simulink model "TestQ"  (R2018b)
settings: Solver=VariableStepAuto  StartTime=0.0  StopTime=tSimEnd  MaxStep=0.001  RelTol=1e-3  EnableMultiTasking=on
InitFcn:
  | clear
  | load 2017-07-18-13-36-00_fullrate_back_forth.mat
  | if ~exist( 'logOriginal' )
  |     logOriginal = dataInOriginal
  | end
  | flog = logOriginal;
  | tSart = flog.vehicle_attitude.time(1);
  | timeStep = 0; % flog.vehicle_attitude.time(2) - flog.vehicle_attitude.time(1);
  | flog.sensor_combined.time = flog.sensor_combined.time - flog.vehicle_attitude.time(1) - timeStep;
  | flog.att_pos_mocap.time = flog.att_pos_mocap.time - flog.vehicle_attitude.time(1) - timeStep;
  | flog.control_state.time = flog.control_state.time - flog.vehicle_attitude.time(1) - timeStep;
  | flog.vehicle_global_position.time = flog.vehicle_global_position.time - flog.vehicle_attitude.time(1) - timeStep;
  | flog.vehicle_attitude.time = flog.vehicle_attitude.time - flog.vehicle_attitude.time(1);
  | 
  | tSimEnd = flog.vehicle_attitude.time(end);
libraries: simulink_extras x3
(part 1 of 2)
settings Model: Creator=jban039  LastModifiedBy=jban039
settings DataIOCC: LimitDataPoints=on
settings OptimizationCC: LifeSpan=inf
settings DebuggingCC: AllowSymbolicDim=off  SFUnexpectedBacktrackingDiag=warning  SFNoUnconditionalDefaultTransitionDiag=warning  SFExecutionAtInitializationDiag=none
settings ModelReferenceCC: PropagateSignalLabelsOutOfModel=off
settings SFSimCC: SimUseLocalCustomCode=off
settings RTWCC: RTWUseLocalCustomCode=off
settings CodeAppCC: StateflowObjectComments=on
settings GRTTargetCC: TargetLangStandard=C89/C90 (ANSI)
settings ConfigComp: CovMetricSettings=dw  CovHtmlReporting=on  CovSaveCumulativeToWorkspaceVar=on  CovSaveSingleToWorkspaceVar=on  CovExternalEMLEnable=off

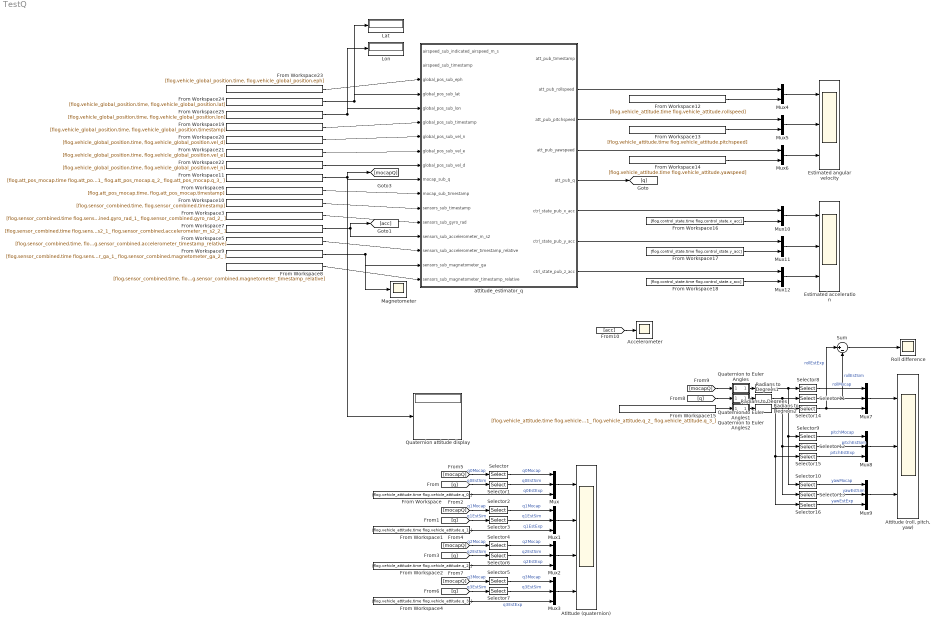
== system TestQ ==
  Accelerometer : Scope
  Atittude (quaternion) : Scope  NumInputPorts=4
  "Attitude (roll, pitch, yaw)" : Scope  NumInputPorts=3
  Estimated acceleration : Scope  NumInputPorts=3
  Estimated angular velocity : Scope  NumInputPorts=3
  From Workspace : FromWorkspace  VariableName=[flog.vehicle_attitude.time flog.vehicle_attitude.q_0_]  SampleTime=0  Interpolate=off  OutputAfterFinalValue=Holding final value
  From Workspace1 : FromWorkspace  VariableName=[flog.vehicle_attitude.time flog.vehicle_attitude.q_1_]  SampleTime=0  Interpolate=off  OutputAfterFinalValue=Holding final value
  From Workspace10 : FromWorkspace  VariableName=[flog.sensor_combined.time, flog.sensor_combined.timestamp]  SampleTime=0  Interpolate=off  OutputAfterFinalValue=Holding final value
  From Workspace11 : FromWorkspace  VariableName=[flog.att_pos_mocap.time flog.att_pos_mocap.q_0_ flog.att_pos_mocap.q_1_ flog.att_pos_mocap.q_2_ flog.att_pos_mocap.q_3_ ]  SampleTime=0  Interpolate=off  OutputAfterFinalValue=Holding final value
  From Workspace12 : FromWorkspace  VariableName=[flog.vehicle_attitude.time flog.vehicle_attitude.rollspeed]  SampleTime=0  Interpolate=off  OutputAfterFinalValue=Holding final value
  From Workspace13 : FromWorkspace  VariableName=[flog.vehicle_attitude.time flog.vehicle_attitude.pitchspeed]  SampleTime=0  Interpolate=off  OutputAfterFinalValue=Holding final value
  From Workspace14 : FromWorkspace  VariableName=[flog.vehicle_attitude.time flog.vehicle_attitude.yawspeed]  SampleTime=0  Interpolate=off  OutputAfterFinalValue=Holding final value
  From Workspace15 : FromWorkspace  VariableName=[flog.vehicle_attitude.time flog.vehicle_attitude.q_0_ flog.vehicle_attitude.q_1_ flog.vehicle_attitude.q_2_ flog.vehicle_attitude.q_3_]  SampleTime=0  Interpolate=off  OutputAfterFinalValue=Holding final value
  From Workspace16 : FromWorkspace  VariableName=[flog.control_state.time flog.control_state.x_acc]  SampleTime=0  Interpolate=off  OutputAfterFinalValue=Holding final value
  From Workspace17 : FromWorkspace  VariableName=[flog.control_state.time flog.control_state.y_acc]  SampleTime=0  Interpolate=off  OutputAfterFinalValue=Holding final value
  From Workspace18 : FromWorkspace  VariableName=[flog.control_state.time flog.control_state.z_acc]  SampleTime=0  Interpolate=off  OutputAfterFinalValue=Holding final value
  From Workspace19 : FromWorkspace  VariableName=[flog.vehicle_global_position.time, flog.vehicle_global_position.timestamp]  SampleTime=0  Interpolate=off  OutputAfterFinalValue=Holding final value
  From Workspace2 : FromWorkspace  VariableName=[flog.vehicle_attitude.time flog.vehicle_attitude.q_2_]  SampleTime=0  Interpolate=off  OutputAfterFinalValue=Holding final value
  From Workspace20 : FromWorkspace  VariableName=[flog.vehicle_global_position.time, flog.vehicle_global_position.vel_d]  SampleTime=0  Interpolate=off  OutputAfterFinalValue=Holding final value
  From Workspace21 : FromWorkspace  VariableName=[flog.vehicle_global_position.time, flog.vehicle_global_position.vel_e]  SampleTime=0  Interpolate=off  OutputAfterFinalValue=Holding final value
  From Workspace22 : FromWorkspace  VariableName=[flog.vehicle_global_position.time, flog.vehicle_global_position.vel_n]  SampleTime=0  Interpolate=off  OutputAfterFinalValue=Holding final value
  From Workspace23 : FromWorkspace  VariableName=[flog.vehicle_global_position.time, flog.vehicle_global_position.eph]  SampleTime=0  Interpolate=off  OutputAfterFinalValue=Holding final value
  From Workspace24 : FromWorkspace  VariableName=[flog.vehicle_global_position.time, flog.vehicle_global_position.lat]  SampleTime=0  Interpolate=off  OutputAfterFinalValue=Holding final value
  From Workspace25 : FromWorkspace  VariableName=[flog.vehicle_global_position.time, flog.vehicle_global_position.lon]  SampleTime=0  Interpolate=off  OutputAfterFinalValue=Holding final value
  From Workspace3 : FromWorkspace  VariableName=[flog.sensor_combined.time flog.sensor_combined.gyro_rad_0_ flog.sensor_combined.gyro_rad_1_ flog.sensor_combined.gyro_rad_2_ ]  SampleTime=0  Interpolate=off  OutputAfterFinalValue=Holding final value
  From Workspace4 : FromWorkspace  VariableName=[flog.vehicle_attitude.time flog.vehicle_attitude.q_3_]  SampleTime=0  Interpolate=off  OutputAfterFinalValue=Holding final value
  From Workspace5 : FromWorkspace  VariableName=[flog.sensor_combined.time, flog.sensor_combined.accelerometer_timestamp_relative]  SampleTime=0  Interpolate=off  OutputAfterFinalValue=Holding final value
  From Workspace6 : FromWorkspace  VariableName=[flog.att_pos_mocap.time, flog.att_pos_mocap.timestamp]  SampleTime=0  Interpolate=off  OutputAfterFinalValue=Holding final value
  From Workspace7 : FromWorkspace  VariableName=[flog.sensor_combined.time flog.sensor_combined.accelerometer_m_s2_0_ flog.sensor_combined.accelerometer_m_s2_1_ flog.sensor_combined.accelerometer_m_s2_2_ ]  SampleTime=0  Interpolate=off  OutputAfterFinalValue=Holding final value
  From Workspace8 : FromWorkspace  VariableName=[flog.sensor_combined.time, flog.sensor_combined.magnetometer_timestamp_relative]  SampleTime=0  Interpolate=off  OutputAfterFinalValue=Holding final value
  From Workspace9 : FromWorkspace  VariableName=[flog.sensor_combined.time flog.sensor_combined.magnetometer_ga_0_ flog.sensor_combined.magnetometer_ga_1_ flog.sensor_combined.magnetometer_ga_2_ ]  SampleTime=0  Interpolate=off  OutputAfterFinalValue=Holding final value
  Lat : Display
  Lon : Display
  Magnetometer : Scope
  Mux{,1..3,7..9} (7 alike) : Mux  Inputs=3
  Mux{4..6,10..12} (6 alike) : Mux  Inputs=2
  Quaternion to Euler Angles : Subsystem  AncestorBlock=QuaternionLibrary/Quaternion to Euler Angles
      mask help: Convert an orientation quaternion to a vector of Euler angles
      mask Help:
      | Convert an orientation quaternion
      | [q1 q2 q3 q4]
      | where:
      | - q1 is the rotation in radians
      | - [q2 q3 q4] is the vector around which the rotation is performed)
      | to a vector of Euler angles
      | [roll, pitch, yaw]
      | Based on code from the PX4 firmware: https://github.com/PX4/Firmware
      mask Display: disp('Q2E')
  Quaternion to Euler Angles1 : Subsystem  AncestorBlock=QuaternionLibrary/Quaternion to Euler Angles
      mask help: Convert an orientation quaternion to a vector of Euler angles
      mask Help:
      | Convert an orientation quaternion
      | [q1 q2 q3 q4]
      | where:
      | - q1 is the rotation in radians
      | - [q2 q3 q4] is the vector around which the rotation is performed)
      | to a vector of Euler angles
      | [roll, pitch, yaw]
      | Based on code from the PX4 firmware: https://github.com/PX4/Firmware
      mask Display: disp('Q2E')
  Quaternion to Euler Angles2 : Subsystem  AncestorBlock=QuaternionLibrary/Quaternion to Euler Angles
      mask help: Convert an orientation quaternion to a vector of Euler angles
      mask Help:
      | Convert an orientation quaternion
      | [q1 q2 q3 q4]
      | where:
      | - q1 is the rotation in radians
      | - [q2 q3 q4] is the vector around which the rotation is performed)
      | to a vector of Euler angles
      | [roll, pitch, yaw]
      | Based on code from the PX4 firmware: https://github.com/PX4/Firmware
      mask Display: disp('Q2E')
  Quaternion attitude display : Display
  Radians to Degrees : simulink_extras/Transformations/Radians to Degrees
  Radians to Degrees1 : simulink_extras/Transformations/Radians to Degrees
  Radians to Degrees2 : simulink_extras/Transformations/Radians to Degrees
  Roll difference : Scope
  Selector : Selector  InputPortWidth=4  IndexOptions=Index vector (dialog)  Indices=[1]  OutputSizes=1
  Selector1 : Selector  InputPortWidth=4  IndexOptions=Index vector (dialog)  Indices=[1]  OutputSizes=1
  Selector10 : Selector  InputPortWidth=3  IndexOptions=Index vector (dialog)  Indices=3  OutputSizes=1
  Selector{8..9,11..12,14..15} (6 alike) : Selector  InputPortWidth=3  IndexOptions=Index vector (dialog)  Indices=[1]  OutputSizes=1
  Selector13 : Selector  InputPortWidth=3  IndexOptions=Index vector (dialog)  Indices=3  OutputSizes=1
  Selector16 : Selector  InputPortWidth=3  IndexOptions=Index vector (dialog)  Indices=3  OutputSizes=1
  Selector2 : Selector  InputPortWidth=4  IndexOptions=Index vector (dialog)  Indices=2  OutputSizes=1
  Selector3 : Selector  InputPortWidth=4  IndexOptions=Index vector (dialog)  Indices=2  OutputSizes=1
  Selector4 : Selector  InputPortWidth=4  IndexOptions=Index vector (dialog)  Indices=3  OutputSizes=1
  Selector5 : Selector  InputPortWidth=4  IndexOptions=Index vector (dialog)  Indices=4  OutputSizes=1
  Selector6 : Selector  InputPortWidth=4  IndexOptions=Index vector (dialog)  Indices=3  OutputSizes=1
  Selector7 : Selector  InputPortWidth=4  IndexOptions=Index vector (dialog)  Indices=4  OutputSizes=1
  Sum : Sum  Inputs=|+-
  attitude_estimator_q : Subsystem  AncestorBlock=Px4Library/attitude_estimator_q  mask(PX4 LPE (local position estimator): local_position_estimator){Q_SAMPLING_PERIOD=1/250, INIT_Q=[-0.726717000000000,-0.00744072000000000,-0.00534285000000000,-0.686876000000000]', ATT_W_ACC=0.2, ATT_W_MAG=0.1, ATT_W_EXT_HDG=0.1, ATT_W_GYRO_BIAS=0.1, ATT_MAG_DECL=0.0, ATT_MAG_DECL_A=1, ATT_EXT_HDG_M=2, ATT_ACC_COMP=1, ATT_BIAS_MAX=0.05, FW_ARSP_MODE=0}
      mask prompts: Q_SAMPLING_PERIOD "Sampling period (s)"; INIT_Q "INIT_Q - Initial UAV orientation - set to 0 to let controller decide (bugged) (-)"; ATT_W_ACC "ATT_W_ACC - Complimentary filter accelerometer weight (-)"; ATT_W_MAG "ATT_W_MAG - Complimentary filter magnetometer weight (-)"; ATT_W_EXT_HDG "ATT_W_EXT_HDG - Complimentary filter external heading weight (-)"; ATT_W_GYRO_BIAS "ATT_W_GYRO_BIAS - Complimentary filter gyroscope bias weight (-)"; ATT_MAG_DECL "ATT_MAG_DECL - Magnetic declination. Not used when GPS available (deg)"; ATT_MAG_DECL_A "ATT_MAG_DECL_A - Automatic GPS based declination compensation (-)"; ATT_EXT_HDG_M "ATT_EXT_HDG_M - External heading usage mode (from Motion capture/Vision) (-), 0 None 1 Vision 2 Motion Capture"; ATT_ACC_COMP "ATT_ACC_COMP - Acceleration compensation based on GPS velocity. (-)"; ATT_BIAS_MAX "ATT_BIAS_MAX - Gyro bias limit (rad/s)"; FW_ARSP_MODE "FW_ARSP_MODE - Method used to publish the airspeed (-), 0 Measured airspeed 1 Vehicle ground speed 2 Airspeed invalid"
      mask TypeOptions ATT_EXT_HDG_M: 0 | 1 | 2
      mask TypeOptions FW_ARSP_MODE: 0 | 1 | 2
  wires:
  Mux1/1 -> Atittude (quaternion)/2
  Mux/1 -> Atittude (quaternion)/1
  Mux2/1 -> Atittude (quaternion)/3
  attitude_estimator_q/5(att_pub_q) -> [q]
  From Workspace/1 -> Mux/3  "q0EstExp"
  Selector1/1 -> Mux/2  "q0EstSim"
  From Workspace11/1 -> Quaternion attitude display/1, [mocapQ], attitude_estimator_q/10(mocap_sub_q)
  From Workspace6/1 -> attitude_estimator_q/11(mocap_sub_timestamp)
  Selector/1 -> Mux/1  "q0Mocap"
  From Workspace7/1 -> attitude_estimator_q/14(sensors_sub_accelerometer_m_s2), [acc]
  From Workspace9/1 -> attitude_estimator_q/16(sensors_sub_magnetometer_ga), Magnetometer/1
  From Workspace3/1 -> attitude_estimator_q/13(sensors_sub_gyro_rad)
  From Workspace1/1 -> Mux1/3  "q1EstExp"
  Selector3/1 -> Mux1/2  "q1EstSim"
  Selector2/1 -> Mux1/1  "q1Mocap"
  From Workspace2/1 -> Mux2/3  "q2EstExp"
  Selector6/1 -> Mux2/2  "q2EstSim"
  Selector4/1 -> Mux2/1  "q2Mocap"
  Mux3/1 -> Atittude (quaternion)/4
  From Workspace4/1 -> Mux3/3  "q3EstExp"
  Selector7/1 -> Mux3/2  "q3EstSim"
  Selector5/1 -> Mux3/1  "q3Mocap"
  [mocapQ] -> Selector/1  "q0Mocap"
  [q] -> Selector1/1  "q0EstSim"
  [mocapQ] -> Selector2/1  "q1Mocap"
  [q] -> Selector3/1  "q1EstSim"
  [mocapQ] -> Selector4/1  "q2Mocap"
  [q] -> Selector6/1  "q2EstSim"
  [mocapQ] -> Selector5/1  "q3Mocap"
  [q] -> Selector7/1  "q3EstSim"
  From Workspace8/1 -> attitude_estimator_q/17(sensors_sub_magnetometer_timestamp_relative)
  From Workspace5/1 -> attitude_estimator_q/15(sensors_sub_accelerometer_timestamp_relative)
  Mux4/1 -> Estimated angular velocity/1
  Mux5/1 -> Estimated angular velocity/2
  Mux6/1 -> Estimated angular velocity/3
  attitude_estimator_q/2(att_pub_rollspeed) -> Mux4/1
  attitude_estimator_q/3(att_pub_pitchspeed) -> Mux5/1
  attitude_estimator_q/4(att_pub_yawspeed) -> Mux6/1
  From Workspace12/1 -> Mux4/2
  From Workspace13/1 -> Mux5/2
  From Workspace14/1 -> Mux6/2
  Quaternion to Euler Angles/1(euler) -> Radians to Degrees/1
  Quaternion to Euler Angles1/1(euler) -> Radians to Degrees1/1
  Mux7/1 -> "Attitude (roll, pitch, yaw)"/1
  Mux8/1 -> "Attitude (roll, pitch, yaw)"/2
  Mux9/1 -> "Attitude (roll, pitch, yaw)"/3
  Selector8/1 -> Mux7/1  "rollMocap"
  Selector11/1 -> Sum/2, Mux7/2  "rollEstSim"
  Selector9/1 -> Mux8/1  "pitchMocap"
  Selector12/1 -> Mux8/2  "pitchEstSim"
  Selector13/1 -> Mux9/2  "yawEstSim"
  Selector10/1 -> Mux9/1  "yawMocap"
  [mocapQ] -> Quaternion to Euler Angles/1(quaternion)
  [q] -> Quaternion to Euler Angles1/1(quaternion)
  From Workspace15/1 -> Quaternion to Euler Angles2/1(quaternion)
  Selector16/1 -> Mux9/3  "yawEstExp"
  Selector15/1 -> Mux8/3  "pitchEstExp"
  Selector14/1 -> Sum/1, Mux7/3  "rollEstExp"
  Radians to Degrees2/1 -> Selector16/1, Selector15/1, Selector14/1
  Radians to Degrees/1 -> Selector10/1, Selector9/1, Selector8/1
  Radians to Degrees1/1 -> Selector13/1, Selector12/1, Selector11/1
  Quaternion to Euler Angles2/1(euler) -> Radians to Degrees2/1
  Sum/1 -> Roll difference/1
  Mux10/1 -> Estimated acceleration/1
  Mux11/1 -> Estimated acceleration/2
  Mux12/1 -> Estimated acceleration/3
  attitude_estimator_q/6(ctrl_state_pub_x_acc) -> Mux10/1
  attitude_estimator_q/7(ctrl_state_pub_y_acc) -> Mux11/1
  attitude_estimator_q/8(ctrl_state_pub_z_acc) -> Mux12/1
  From Workspace16/1 -> Mux10/2
  From Workspace17/1 -> Mux11/2
  From Workspace18/1 -> Mux12/2
  From Workspace10/1 -> attitude_estimator_q/12(sensors_sub_timestamp)
  From Workspace20/1 -> attitude_estimator_q/7(global_pos_sub_vel_n)
  From Workspace19/1 -> attitude_estimator_q/6(global_pos_sub_timestamp)
  From Workspace21/1 -> attitude_estimator_q/8(global_pos_sub_vel_e)
  From Workspace22/1 -> attitude_estimator_q/9(global_pos_sub_vel_d)
  From Workspace25/1 -> attitude_estimator_q/5(global_pos_sub_lon), Lon/1
  From Workspace24/1 -> attitude_estimator_q/4(global_pos_sub_lat), Lat/1
  From Workspace23/1 -> attitude_estimator_q/3(global_pos_sub_eph)
  [acc] -> Accelerometer/1

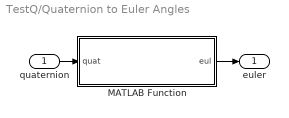
== system TestQ/Quaternion to Euler Angles ==
  quaternion : Inport
  MATLAB Function : MATLAB Function  TreatAsAtomicUnit=on
  euler : Outport
  wires:
  quaternion/1 -> MATLAB Function/1(quat)
  MATLAB Function/1(eul) -> euler/1

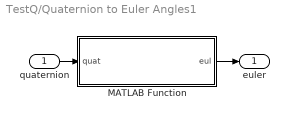
== system TestQ/Quaternion to Euler Angles1 ==
  quaternion : Inport
  MATLAB Function : MATLAB Function  TreatAsAtomicUnit=on
  euler : Outport
  wires:
  quaternion/1 -> MATLAB Function/1(quat)
  MATLAB Function/1(eul) -> euler/1

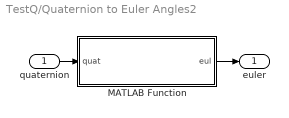
== system TestQ/Quaternion to Euler Angles2 ==
  quaternion : Inport
  MATLAB Function : MATLAB Function  TreatAsAtomicUnit=on
  euler : Outport
  wires:
  quaternion/1 -> MATLAB Function/1(quat)
  MATLAB Function/1(eul) -> euler/1

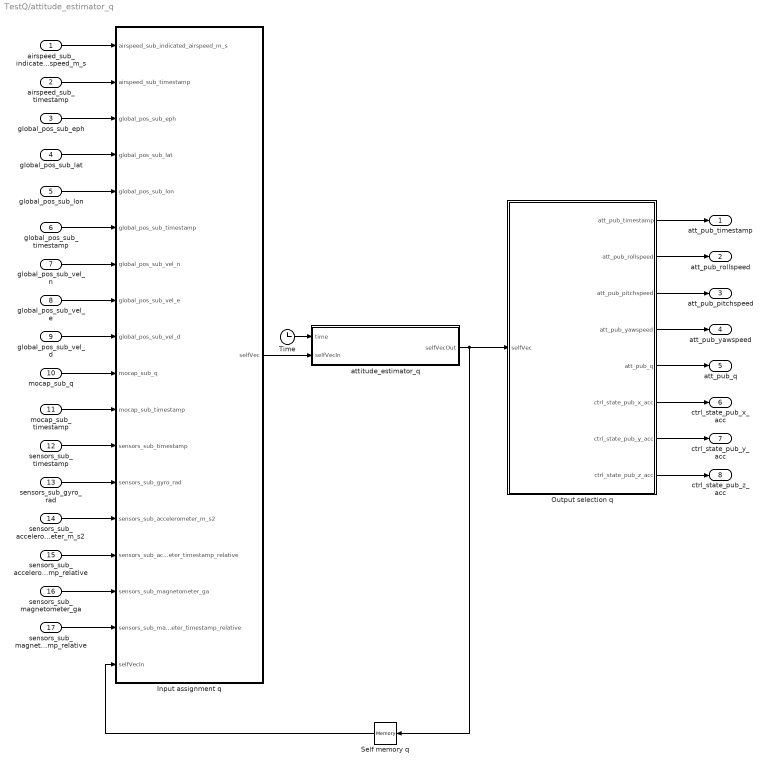
== system TestQ/attitude_estimator_q ==
  airspeed_sub_indicated_airspeed_m_s : Inport
  airspeed_sub_timestamp : Inport  Port=2
  global_pos_sub_eph : Inport  Port=3
  global_pos_sub_lat : Inport  Port=4
  global_pos_sub_lon : Inport  Port=5
  global_pos_sub_timestamp : Inport  Port=6
  global_pos_sub_vel_n : Inport  Port=7
  global_pos_sub_vel_e : Inport  Port=8
  global_pos_sub_vel_d : Inport  Port=9
  mocap_sub_q : Inport  Port=10
  mocap_sub_timestamp : Inport  Port=11
  sensors_sub_timestamp : Inport  Port=12
  sensors_sub_gyro_rad : Inport  Port=13
  sensors_sub_accelerometer_m_s2 : Inport  Port=14
  sensors_sub_accelerometer_timestamp_relative : Inport  Port=15
  sensors_sub_magnetometer_ga : Inport  Port=16
  sensors_sub_magnetometer_timestamp_relative : Inport  Port=17
  Input assignment q : MATLAB Function  TreatAsAtomicUnit=on
  Output selection q : MATLAB Function  TreatAsAtomicUnit=on
  Self memory q : Memory  InitialCondition=[ATT_ACC_COMP, 0, 0, 0, 0, 0, 0, 0, FW_ARSP_MODE, 0, 0, 0, 0, 0, 0, 0, 0, INIT_Q(1), INIT_Q(2), INIT_Q(3), INIT_Q(4), ATT_BIAS_MAX, 0, 0, INIT_Q(1), INIT_Q(2), INIT_Q(3), INIT_Q(4), 0, 0, 0, 0, 0, 0, 0, 0, 0, 0, 0, 0, 0.02, 0, ATT_EXT_HDG_M, 0, 0, 0, 0, 0, 0, 0, 0, 0, 0, 0, 0, 0, 0, 0, 0, 0, 0, 0, 0, 0, 0, 0, 0, 0, 0, 0, 0, 0, 0, 0, 0, 0, 0, 0, 0, 0, 0, 0, 0, 0, 0, 0, 0, 0, 0, 0, 0, 0, 0, 0, 0, 0, 0, 0, 0, 0, 0, 0, 0, 0, 0, 0, 0, 0, 0, 0, 0, 0, 0, 0, 0, 0, 0, 0, 0, 0, 0, 0, 0, 0, 0, 0, 0, 0, 0, 0, 0, 0, ATT_MAG_DECL, ATT_MAG_DECL_A, 0, 0, 0, 0, 0, 0, 0, 0, 0, 0, 0, 0, 0, 0, 0, 0, 0, 0, 0, 0, 0, 0, INIT_Q(1), INIT_Q(2), INIT_Q(3), INIT_Q(4), 0, 0, 0, 0, 0, 0, 0, 0, 0, 0, 0, 0, 0, 0, 0, 0, 0, 0, 0, 0, 0, 0, 0, 0, 0, 0, 0, 0, 0, 0, 0, 0, 0, 0, 0, 0, 0, 0, 0, ATT_W_ACC, ATT_W_EXT_HDG, ATT_W_GYRO_BIAS, ATT_W_MAG, 0, 0]
  Time : Clock
  attitude_estimator_q : MATLAB Function  TreatAsAtomicUnit=on  SystemSampleTime=Q_SAMPLING_PERIOD
  att_pub_timestamp : Outport
  att_pub_rollspeed : Outport  Port=2
  att_pub_pitchspeed : Outport  Port=3
  att_pub_yawspeed : Outport  Port=4
  att_pub_q : Outport  Port=5
  ctrl_state_pub_x_acc : Outport  Port=6
  ctrl_state_pub_y_acc : Outport  Port=7
  ctrl_state_pub_z_acc : Outport  Port=8
  wires:
  Output selection q/8(ctrl_state_pub_z_acc) -> ctrl_state_pub_z_acc/1
  Output selection q/7(ctrl_state_pub_y_acc) -> ctrl_state_pub_y_acc/1
  Output selection q/6(ctrl_state_pub_x_acc) -> ctrl_state_pub_x_acc/1
  Output selection q/5(att_pub_q) -> att_pub_q/1
  Output selection q/4(att_pub_yawspeed) -> att_pub_yawspeed/1
  Output selection q/3(att_pub_pitchspeed) -> att_pub_pitchspeed/1
  Output selection q/2(att_pub_rollspeed) -> att_pub_rollspeed/1
  Output selection q/1(att_pub_timestamp) -> att_pub_timestamp/1
  sensors_sub_magnetometer_timestamp_relative/1 -> Input assignment q/17(sensors_sub_magnetometer_timestamp_relative)
  sensors_sub_magnetometer_ga/1 -> Input assignment q/16(sensors_sub_magnetometer_ga)
  sensors_sub_accelerometer_timestamp_relative/1 -> Input assignment q/15(sensors_sub_accelerometer_timestamp_relative)
  sensors_sub_accelerometer_m_s2/1 -> Input assignment q/14(sensors_sub_accelerometer_m_s2)
  sensors_sub_gyro_rad/1 -> Input assignment q/13(sensors_sub_gyro_rad)
  sensors_sub_timestamp/1 -> Input assignment q/12(sensors_sub_timestamp)
  mocap_sub_timestamp/1 -> Input assignment q/11(mocap_sub_timestamp)
  mocap_sub_q/1 -> Input assignment q/10(mocap_sub_q)
  global_pos_sub_vel_d/1 -> Input assignment q/9(global_pos_sub_vel_d)
  global_pos_sub_vel_e/1 -> Input assignment q/8(global_pos_sub_vel_e)
  global_pos_sub_vel_n/1 -> Input assignment q/7(global_pos_sub_vel_n)
  global_pos_sub_timestamp/1 -> Input assignment q/6(global_pos_sub_timestamp)
  global_pos_sub_lon/1 -> Input assignment q/5(global_pos_sub_lon)
  global_pos_sub_lat/1 -> Input assignment q/4(global_pos_sub_lat)
  global_pos_sub_eph/1 -> Input assignment q/3(global_pos_sub_eph)
  airspeed_sub_timestamp/1 -> Input assignment q/2(airspeed_sub_timestamp)
  airspeed_sub_indicated_airspeed_m_s/1 -> Input assignment q/1(airspeed_sub_indicated_airspeed_m_s)
  Time/1 -> attitude_estimator_q/1(time)
  Self memory q/1 -> Input assignment q/18(selfVecIn)
  attitude_estimator_q/1(selfVecOut) -> Self memory q/1, Output selection q/1(selfVec)
  Input assignment q/1(selfVec) -> attitude_estimator_q/2(selfVecIn)

== matlab function TestQ/Quaternion to Euler Angles1/MATLAB Function ==
  data: quat input; eul output
function eul   = QuaternionToEuler( quat )
%QUATERNIONTOEULER Convert quaternion to euler angles
%   Based on PX4 Firmware code: https://github.com/PX4/Firmware
%   Written by:    J.X.J. Bannwarth, 2016/08/29
%   Last modified: J.X.J. Bannwarth, 2018/12/11

    eul = [ atan2(2.0 .* (quat(1) .* quat(2) + quat(3) .* quat(4)), ...
                1.0 - 2.0 .* (quat(2) .* quat(2) + quat(3) .* quat(3)));
	        asin(2.0 .* (quat(1) .* quat(3) - quat(4) .* quat(2)));
            atan2(2.0 .* (quat(1) .* quat(4) + quat(2) .* quat(3)), ...
                1.0 - 2.0 .* (quat(3) .* quat(3) + quat(4) .* quat(4))) ];
end

== matlab function TestQ/Quaternion to Euler Angles/MATLAB Function ==
  data: quat input; eul output
function eul   = QuaternionToEuler( quat )
%QUATERNIONTOEULER Convert quaternion to euler angles
%   Based on PX4 Firmware code: https://github.com/PX4/Firmware
%   Written by:    J.X.J. Bannwarth, 2016/08/29
%   Last modified: J.X.J. Bannwarth, 2018/12/11

    eul = [ atan2(2.0 .* (quat(1) .* quat(2) + quat(3) .* quat(4)), ...
                1.0 - 2.0 .* (quat(2) .* quat(2) + quat(3) .* quat(3)));
	        asin(2.0 .* (quat(1) .* quat(3) - quat(4) .* quat(2)));
            atan2(2.0 .* (quat(1) .* quat(4) + quat(2) .* quat(3)), ...
                1.0 - 2.0 .* (quat(3) .* quat(3) + quat(4) .* quat(4))) ];
end

== matlab function TestQ/Quaternion to Euler Angles2/MATLAB Function ==
  data: quat input; eul output
function eul   = QuaternionToEuler( quat )
%QUATERNIONTOEULER Convert quaternion to euler angles
%   Based on PX4 Firmware code: https://github.com/PX4/Firmware
%   Written by:    J.X.J. Bannwarth, 2016/08/29
%   Last modified: J.X.J. Bannwarth, 2018/12/11

    eul = [ atan2(2.0 .* (quat(1) .* quat(2) + quat(3) .* quat(4)), ...
                1.0 - 2.0 .* (quat(2) .* quat(2) + quat(3) .* quat(3)));
	        asin(2.0 .* (quat(1) .* quat(3) - quat(4) .* quat(2)));
            atan2(2.0 .* (quat(1) .* quat(4) + quat(2) .* quat(3)), ...
                1.0 - 2.0 .* (quat(3) .* quat(3) + quat(4) .* quat(4))) ];
end

== matlab function TestQ/attitude_estimator_q/Input assignment q ==
  data: airspeed_sub_indicated_airspeed_m_s input; airspeed_sub_timestamp input; global_pos_sub_eph input; global_pos_sub_lat input; global_pos_sub_lon input; global_pos_sub_timestamp input; global_pos_sub_vel_n input; global_pos_sub_vel_e input; global_pos_sub_vel_d input; mocap_sub_q input; mocap_sub_timestamp input; sensors_sub_timestamp input; sensors_sub_gyro_rad input; sensors_sub_accelerometer_m_s2 input; sensors_sub_accelerometer_timestamp_relative input; sensors_sub_magnetometer_ga input; sensors_sub_magnetometer_timestamp_relative input; selfVecIn input; selfVec output
function selfVec = InputAssignment( ...
	     airspeed_sub_indicated_airspeed_m_s, ...
	                  airspeed_sub_timestamp, ...
	                      global_pos_sub_eph, ...
	                      global_pos_sub_lat, ...
	                      global_pos_sub_lon, ...
	                global_pos_sub_timestamp, ...
	                    global_pos_sub_vel_n, ...
	                    global_pos_sub_vel_e, ...
	                    global_pos_sub_vel_d, ...
	                             mocap_sub_q, ...
	                     mocap_sub_timestamp, ...
	                   sensors_sub_timestamp, ...
	                    sensors_sub_gyro_rad, ...
	          sensors_sub_accelerometer_m_s2, ...
	sensors_sub_accelerometer_timestamp_relative, ...
	             sensors_sub_magnetometer_ga, ...
	sensors_sub_magnetometer_timestamp_relative, ...
	                               selfVecIn ...
	)
%#codegen

	selfVec = selfVecIn;

	% Variable assignment
	selfVec(10:10) =      airspeed_sub_indicated_airspeed_m_s;
	selfVec(11:11) =                   airspeed_sub_timestamp;
	selfVec(45:45) =                       global_pos_sub_eph;
	selfVec(46:46) =                       global_pos_sub_lat;
	selfVec(47:47) =                       global_pos_sub_lon;
	selfVec(48:48) =                 global_pos_sub_timestamp;
	selfVec(50:50) =                     global_pos_sub_vel_n;
	selfVec(51:51) =                     global_pos_sub_vel_e;
	selfVec(52:52) =                     global_pos_sub_vel_d;
	selfVec(147:150) =                              mocap_sub_q;
	selfVec(151:151) =                      mocap_sub_timestamp;
	selfVec(166:166) =                    sensors_sub_timestamp;
	selfVec(168:170) =                     sensors_sub_gyro_rad;
	selfVec(171:173) =           sensors_sub_accelerometer_m_s2;
	selfVec(174:174) = sensors_sub_accelerometer_timestamp_relative;
	selfVec(175:177) =              sensors_sub_magnetometer_ga;
	selfVec(178:178) = sensors_sub_magnetometer_timestamp_relative;
end

== matlab function TestQ/attitude_estimator_q/Output selection q ==
  data: att_pub_timestamp output; att_pub_rollspeed output; att_pub_pitchspeed output; att_pub_yawspeed output; att_pub_q output; selfVec input; ctrl_state_pub_x_acc output; ctrl_state_pub_y_acc output; ctrl_state_pub_z_acc output
function [ ...
                        att_pub_timestamp, ...
                        att_pub_rollspeed, ...
                       att_pub_pitchspeed, ...
                         att_pub_yawspeed, ...
                                att_pub_q, ...
                     ctrl_state_pub_x_acc, ...
                     ctrl_state_pub_y_acc, ...
                     ctrl_state_pub_z_acc] ...
   = OutputSelection( selfVec )
%#codegen

	% Variable assignment
	                       att_pub_timestamp = selfVec(14:14);
	                       att_pub_rollspeed = selfVec(15:15);
	                      att_pub_pitchspeed = selfVec(16:16);
	                        att_pub_yawspeed = selfVec(17:17);
	                               att_pub_q = selfVec(18:21);
	                    ctrl_state_pub_x_acc = selfVec(29:29);
	                    ctrl_state_pub_y_acc = selfVec(30:30);
	                    ctrl_state_pub_z_acc = selfVec(31:31);
end
